simulink model "pid_regler"  (Simulink 4.00)
settings: Solver=ode45  StartTime=0.0  StopTime=10.0  RelTol=1e-3
values from neighbouring files (symbols this model uses):
  N = 5    [anw_pid_1.m]    (also in inv_switch_1.m = 200)
  Td = 80    [anw_pid_1.m]
settings Model: LastModifiedBy=Administrator  BlockReductionOpt=off

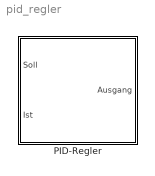
== system pid_regler ==
  PID-Regler : Subsystem
      settings: RTWFcnNameOpts=Auto  RTWFileNameOpts=Auto

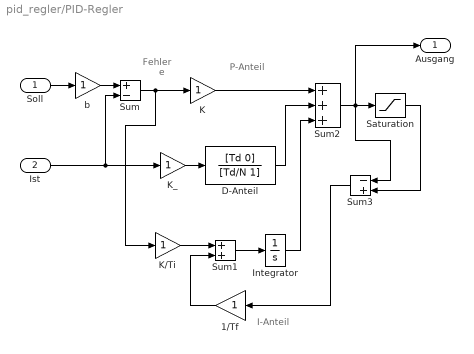
== system pid_regler/PID-Regler ==
  note: P-Anteil
  note: Fehler
  note: e
  note: I-Anteil
  Soll : Inport  Port=1
  Ist : Inport  Port=2
  1/Tf : Gain  Orientation=left  Gain=1  Multiplication=Element-wise(K.*u)  SaturateOnIntegerOverflow=on
  "D-Anteil " : TransferFcn  Numerator=[Td 0]  Denominator=[Td/N 1]  Realization=auto  AbsoluteTolerance=auto
  Integrator : Integrator  ExternalReset=none  InitialConditionSource=internal  InitialCondition=0  LimitOutput=off  UpperSaturationLimit=inf  LowerSaturationLimit=-inf  ShowSaturationPort=off  ShowStatePort=off  AbsoluteTolerance=auto
  K : Gain  Gain=1  Multiplication=Element-wise(K.*u)  SaturateOnIntegerOverflow=on
  K/Ti : Gain  Gain=1  Multiplication=Element-wise(K.*u)  SaturateOnIntegerOverflow=on
  K_ : Gain  Gain=1  Multiplication=Element-wise(K.*u)  SaturateOnIntegerOverflow=on
  Saturation : Saturate  UpperLimit=0.5  LowerLimit=-0.5  LinearizeAsGain=on
  Sum : Sum  Inputs=+-  SaturateOnIntegerOverflow=on
  Sum1 : Sum  Inputs=++  SaturateOnIntegerOverflow=on
  Sum2 : Sum  Inputs=+++  SaturateOnIntegerOverflow=on
  Sum3 : Sum  Orientation=left  Inputs=-+  SaturateOnIntegerOverflow=on
  b : Gain  Gain=1  Multiplication=Element-wise(K.*u)  SaturateOnIntegerOverflow=on
  Ausgang : Outport  Port=1
  wires:
  Ist/1 -> K_/1, Sum/2
  Soll/1 -> b/1
  Sum3/1 -> 1/Tf/1
  1/Tf/1 -> Sum1/2
  Sum/1 -> K/Ti/1, K/1
  K/Ti/1 -> Sum1/1
  Sum1/1 -> Integrator/1
  Integrator/1 -> Sum2/3
  "D-Anteil "/1 -> Sum2/2
  K_/1 -> "D-Anteil "/1
  b/1 -> Sum/1
  K/1 -> Sum2/1
  Saturation/1 -> Sum3/2
  Sum2/1 -> Ausgang/1, Sum3/1, Saturation/1
